simulink model "modified_DDPG_ACC"  (R2021b)
settings: Solver=FixedStepAuto  StartTime=0.0  StopTime=Inf  RelTol=1e-3
values from neighbouring files (symbols this model uses):
  amax_ego = 3    [ACC_Integration.m]
  amin_ego = -3    [ACC_Integration.m]
  t_gap = 1.4    [ACC_Integration.m]
  Ts = 0.1    [ACC_Integration.m]
  v0_ego = 0    [ACC_Integration.m]
  v0_lead = 0    [ACC_Integration.m]
  v_max_ego = 66.6    [ACC_Integration.m]
  v_max_lead = 66.6    [ACC_Integration.m]
  v_min_ego = 0    [ACC_Integration.m]
  v_min_lead = 0    [ACC_Integration.m]
  v_set = 30    [ACC_Integration.m]
  x0_ego = 10    [ACC_Integration.m]
  x0_lead = 50    [ACC_Integration.m]
libraries: simulink x2, mpcadaslib x1, rllib x1
settings Model: Creator=The MathWorks, Inc.  LastModifiedBy=Niklas
settings SolverCC: AlgebraicLoopSolver=TrustRegion
settings DebuggingCC: SFMachineParentedDataDiag=warning  ArithmeticOperatorsInVariantConditions=warning
settings SFSimCC: SimUseLocalCustomCode=off
settings RTWCC: RTWUseLocalCustomCode=off
settings CodeAppCC: StateflowObjectComments=on

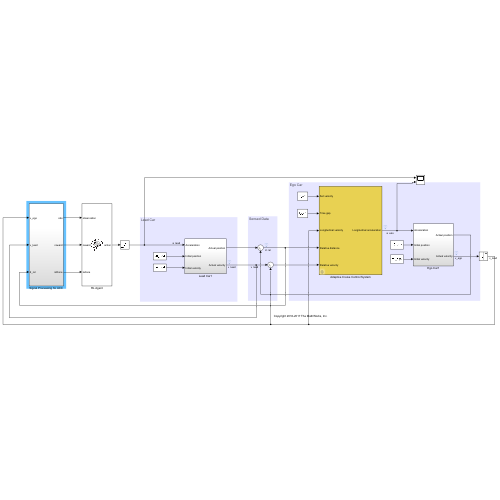
[thumbnail: Simulink's stored preview of the top-level diagram]
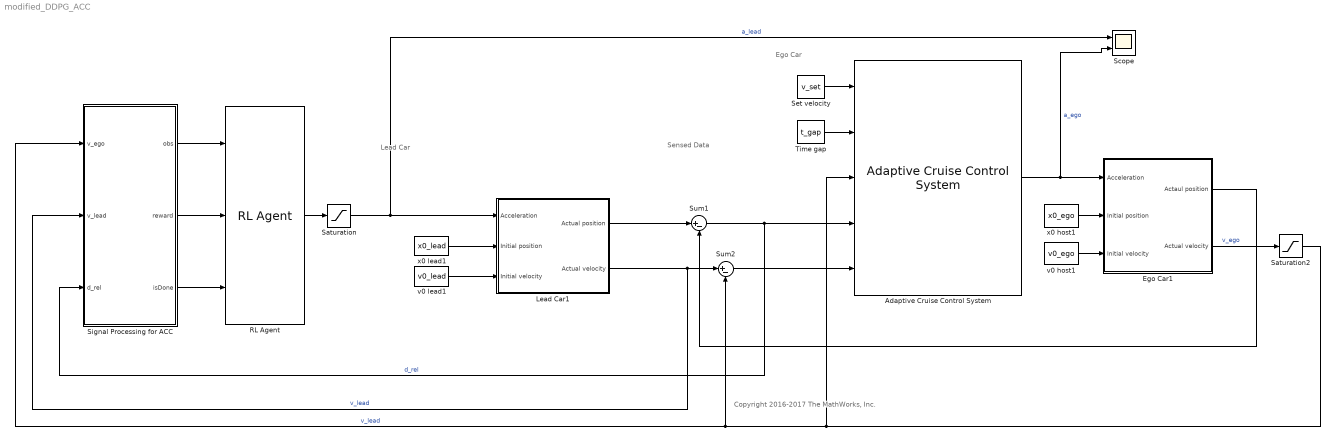
== system modified_DDPG_ACC ==
  note: Sensed Data
  note: Ego Car
  note: Lead Car
  note: Copyright 2016-2017 The MathWorks, Inc.
  Adaptive Cruise Control System : mpcadaslib/Adaptive Cruise Control System  EgoModel=tf(1,[0.5,1,0])  InitialEgoVelocity=20  DefaultSpacing=0  MaxVelocity=50  MinAcceleration=-3  amin_ext=off  MaxAcceleration=3  amax_ext=off  Ts=0.1  PredictionHorizon=30  ControllerBehavior=0.5  suboptimal=off  maxiter=10  datatypeopt=double  optmode=off  trackmode=off
  Ego Car1 : Subsystem
  Lead Car1 : Subsystem
  RL Agent : rllib/RL Agent  Agent=agent  ExternalActionAsInput=off  ProvideCumRwd=off  TreatAsDirectFeedthrough=on
      settings: SourceProductName=Reinforcement Learning
  Saturation : Saturate  UpperLimit=amax_ego  LowerLimit=amin_ego
  Saturation2 : Saturate  UpperLimit=v_max_ego  LowerLimit=v_min_ego
  Scope : Scope  NumInputPorts=2
  Set velocity : Constant  Value=v_set  SampleTime=Ts
  Signal Processing for ACC : Subsystem
  Sum1 : Sum  Inputs=|+-
  Sum2 : Sum  Inputs=|+-
  Time gap : Constant  Value=t_gap  SampleTime=Ts
  v0 host1 : Constant  Value=v0_ego  SampleTime=Ts
  v0 lead1 : Constant  Value=v0_lead  SampleTime=Ts
  x0 host1 : Constant  Value=x0_ego  SampleTime=Ts
  x0 lead1 : Constant  Value=x0_lead  SampleTime=Ts
  wires:
  Signal Processing for ACC/2(reward) -> RL Agent/2
  RL Agent/1 -> Saturation/1
  Signal Processing for ACC/3(isDone) -> RL Agent/3
  Signal Processing for ACC/1(obs) -> RL Agent/1
  Sum2/1 -> Adaptive Cruise Control System/5
  Time gap/1 -> Adaptive Cruise Control System/2
  Saturation/1 -> Scope/1, Lead Car1/1(Acceleration)  "a_lead"
  Sum1/1 -> Signal Processing for ACC/3(d_rel), Adaptive Cruise Control System/4  "d_rel"
  Lead Car1/1(Actual position) -> Sum1/1
  Set velocity/1 -> Adaptive Cruise Control System/1
  v0 lead1/1 -> Lead Car1/3(Initial velocity)
  Ego Car1/1(Actaul position) -> Sum1/2
  v0 host1/1 -> Ego Car1/3(Initial velocity)
  x0 lead1/1 -> Lead Car1/2(Initial position)
  Adaptive Cruise Control System/1 -> Scope/2, Ego Car1/1(Acceleration)  "a_ego"
  x0 host1/1 -> Ego Car1/2(Initial position)
  Lead Car1/2(Actual velocity) -> Signal Processing for ACC/2(v_lead), Sum2/1  "v_lead"
  Ego Car1/2(Actual velocity) -> Saturation2/1  "v_ego"
  Saturation2/1 -> Adaptive Cruise Control System/3, Signal Processing for ACC/1(v_ego), Sum2/2  "v_lead"

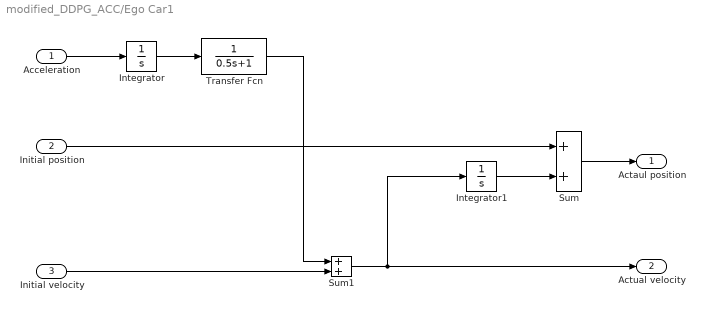
== system modified_DDPG_ACC/Ego Car1 ==
  Acceleration : Inport
  Initial position : Inport  Port=2
  Initial velocity : Inport  Port=3
  Integrator : Integrator
  Integrator1 : Integrator
  Sum : Sum
  Sum1 : Sum
  Transfer Fcn : TransferFcn  Denominator=[0.5 1]
  Actaul position : Outport  VectorParamsAs1DForOutWhenUnconnected=off
  Actual velocity : Outport  Port=2  VectorParamsAs1DForOutWhenUnconnected=off
  wires:
  Sum1/1 -> Integrator1/1, Actual velocity/1
  Initial velocity/1 -> Sum1/2
  Sum/1 -> Actaul position/1
  Transfer Fcn/1 -> Sum1/1
  Integrator/1 -> Transfer Fcn/1
  Acceleration/1 -> Integrator/1
  Initial position/1 -> Sum/1
  Integrator1/1 -> Sum/2

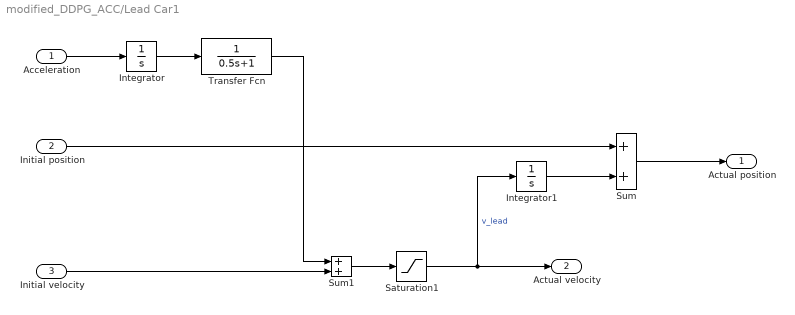
== system modified_DDPG_ACC/Lead Car1 ==
  Acceleration : Inport
  Initial position : Inport  Port=2
  Initial velocity : Inport  Port=3
  Integrator : Integrator
  Integrator1 : Integrator
  Saturation1 : Saturate  UpperLimit=v_max_lead  LowerLimit=v_min_lead
  Sum : Sum
  Sum1 : Sum
  Transfer Fcn : TransferFcn  Denominator=[0.5 1]
  Actual position : Outport  VectorParamsAs1DForOutWhenUnconnected=off
  Actual velocity : Outport  Port=2  VectorParamsAs1DForOutWhenUnconnected=off
  wires:
  Transfer Fcn/1 -> Sum1/1
  Initial velocity/1 -> Sum1/2
  Sum/1 -> Actual position/1
  Integrator/1 -> Transfer Fcn/1
  Sum1/1 -> Saturation1/1
  Acceleration/1 -> Integrator/1
  Initial position/1 -> Sum/1
  Integrator1/1 -> Sum/2
  Saturation1/1 -> Integrator1/1, Actual velocity/1  "v_lead"

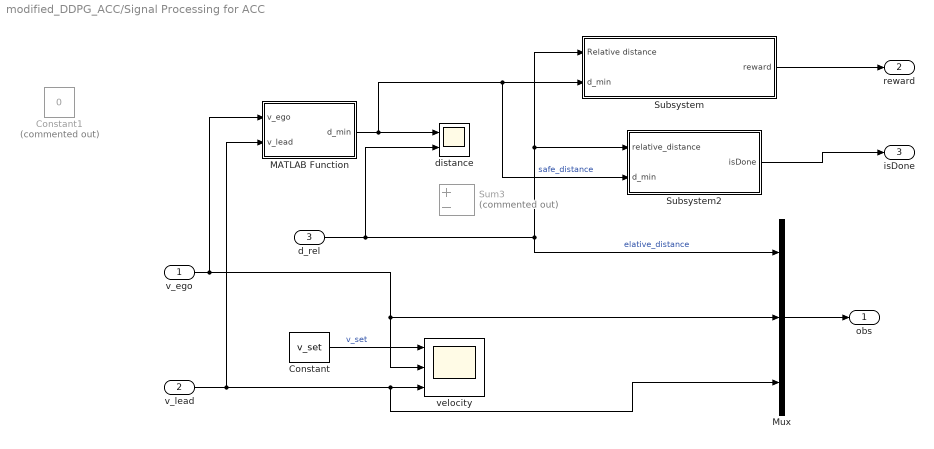
== system modified_DDPG_ACC/Signal Processing for ACC ==
  v_ego : Inport
  v_lead : Inport  Port=2
  d_rel : Inport  Port=3
  Constant : Constant  Value=v_set
  Constant1 : Constant  Commented=on  Value=0
  MATLAB Function : MATLAB Function  TreatAsAtomicUnit=on
  Mux : Mux  Inputs=3
  Subsystem : Subsystem
  Subsystem2 : Subsystem
  Sum3 : Sum  Commented=on  Inputs=+-
  distance : Scope  NumInputPorts=2
  velocity : Scope  NumInputPorts=3
  obs : Outport  VectorParamsAs1DForOutWhenUnconnected=off
  reward : Outport  Port=2  VectorParamsAs1DForOutWhenUnconnected=off
  isDone : Outport  Port=3  VectorParamsAs1DForOutWhenUnconnected=off
  wires:
  Constant/1 -> velocity/1  "v_set"
  v_lead/1 -> Mux/3, velocity/3, MATLAB Function/2(v_lead)
  Mux/1 -> obs/1
  v_ego/1 -> MATLAB Function/1(v_ego), velocity/2, Mux/2
  d_rel/1 -> distance/2, Mux/1, Subsystem/1(Relative distance), Subsystem2/1(relative_distance)  "elative_distance"
  Subsystem2/1(isDone) -> isDone/1
  Subsystem/1(reward) -> reward/1
  MATLAB Function/1(d_min) -> Subsystem2/2(d_min), Subsystem/2(d_min), distance/1  "safe_distance"

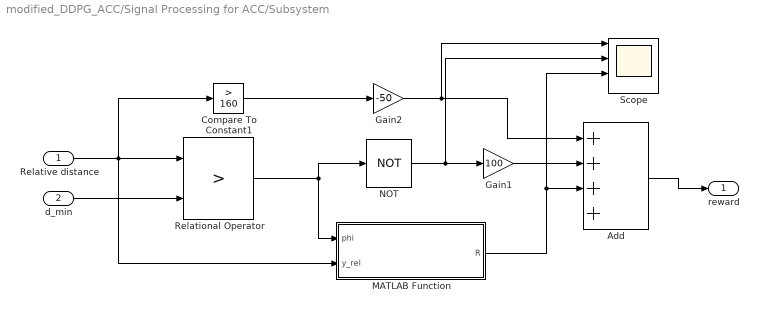
== system modified_DDPG_ACC/Signal Processing for ACC/Subsystem ==
  Relative distance : Inport
  d_min : Inport  Port=2
  Add : Sum  Inputs=++++
  Compare To Constant1 : simulink/Logic and Bit Operations/Compare To Constant  relop=>  const=160  OutDataTypeStr=boolean
  Gain1 : Gain  Gain=100
  Gain2 : Gain  Gain=-50
  MATLAB Function : MATLAB Function  TreatAsAtomicUnit=on
  NOT : Logic  Operator=NOT  IconShape=distinctive  AllPortsSameDT=off  OutDataTypeStr=boolean
  Relational Operator : RelationalOperator  Operator=>  OutDataTypeStr=boolean  RndMeth=Simplest
  Scope : Scope  NumInputPorts=4
  reward : Outport
  wires:
  Relative distance/1 -> Compare To Constant1/1, Relational Operator/1, MATLAB Function/2(y_rel)
  d_min/1 -> Relational Operator/2
  Relational Operator/1 -> NOT/1, MATLAB Function/1(phi)
  Add/1 -> reward/1
  MATLAB Function/1(R) -> Scope/3, Add/3
  NOT/1 -> Scope/2, Gain1/1
  Gain1/1 -> Add/2
  Compare To Constant1/1 -> Gain2/1
  Gain2/1 -> Scope/1, Add/1

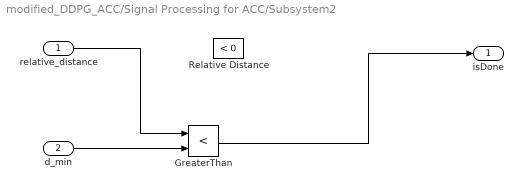
== system modified_DDPG_ACC/Signal Processing for ACC/Subsystem2 ==
  relative_distance : Inport
  d_min : Inport  Port=2
  GreaterThan : RelationalOperator  Operator=<  OutDataTypeStr=boolean  RndMeth=Simplest
  Relative Distance : simulink/Logic and Bit Operations/Compare To Constant  relop=<  const=0  OutDataTypeStr=boolean
  isDone : Outport  VectorParamsAs1DForOutWhenUnconnected=off
  wires:
  relative_distance/1 -> GreaterThan/1
  GreaterThan/1 -> isDone/1
  d_min/1 -> GreaterThan/2

== matlab function modified_DDPG_ACC/Signal Processing for ACC/MATLAB Function ==
  data: v_ego input; d_min output; v_lead input
function d_min=dmin(v_ego,v_lead)
%To compute the minimum distance
% Response time
tr=0.1;
% Max acceleration of ego car 
a_max_acc=3;
% Max acceleration of lead car to full stop
a_max_brake=3;
% Min acceleration of lead car to full stop
a_min_brake=2.5;
temp=v_ego*tr+a_max_acc*tr^2/2 + (v_ego+a_max_acc*tr)^2/(2*a_min_brake) -v_lead^2/(2*a_max_brake);
if temp <0
   d_min=0;
else
   d_min=temp ;
end
end

== matlab function modified_DDPG_ACC/Signal Processing for ACC/Subsystem/MATLAB Function ==
  data: phi input; R output; y_rel input
function R = reward_function(phi, y_rel)
    k = 0.001;
    R = exp(-k*phi*y_rel)-1;
end
